simulink model "BPSK_modulation_demodulation_0"  (R2024a)
settings: Solver=VariableStepAuto  StartTime=0.0  StopTime=0.1  RelTol=1e-3
undefined symbols (not defined in the file or in its folder): Fs, ip, usb
libraries: commdigbbndpm3 x3, dspfdesign x3, commrflib2 x3, commfilt2 x3, dspsigops x3, plutoradiolib x1, simulink x1, dspxfrm3 x1, sdrrlib x1
settings Model: Creator=opr  LastModifiedBy=digital

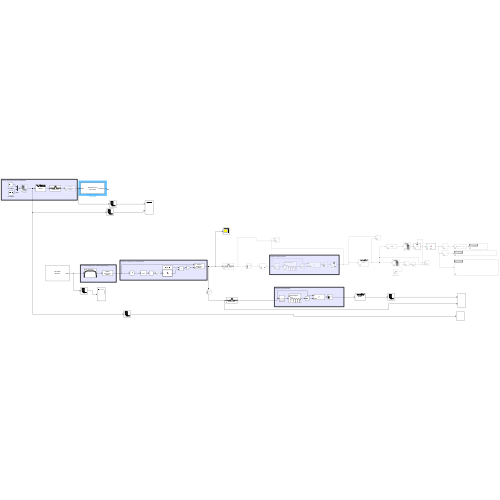
[thumbnail: Simulink's stored preview of the top-level diagram]
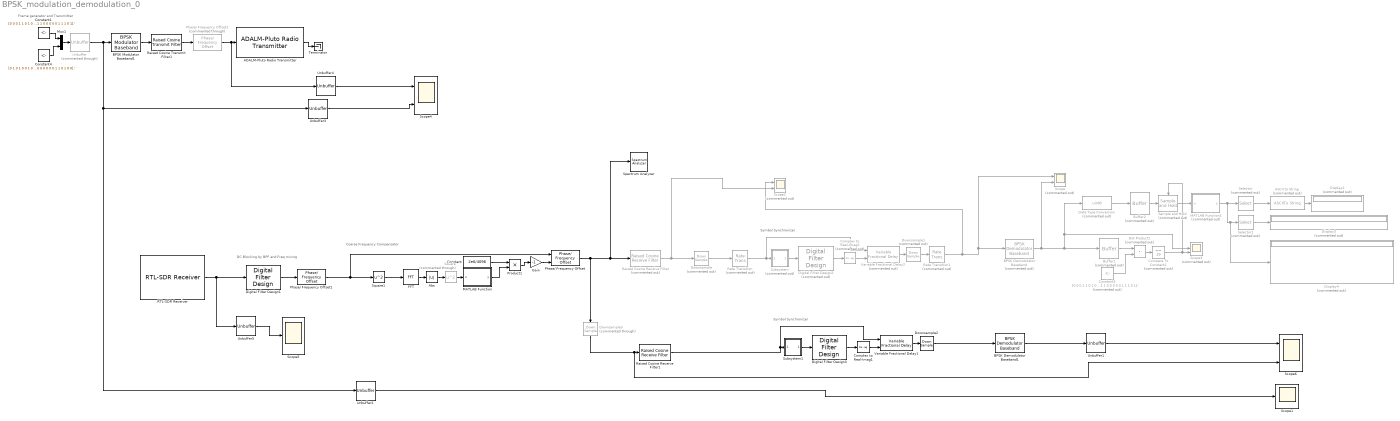
== system BPSK_modulation_demodulation_0 ==
  note: Coarse Frequency Compensator
  note: Frame generator and Transmitter
  note: DC Blocking by BPF and Freq mixing
  note: Symbol Synchronizer
  note: Symbol Synchronizer
  ADALM-Pluto Radio Transmitter : plutoradiolib/ADALM-Pluto Radio Transmitter  RadioID=usb:0  uri=ip:10.0.0.200  CenterFrequencySource=Dialog  CenterFrequency=450e6  GainSource=Dialog  Gain=-30  ChannelMapping=1  BasebandSampleRate=2e6  UnderflowOutputPort=on  ShowAdvancedProperties=off  UseCustomFilter=off  filtPathRates=[737280000 11520000 3840000 1920000 960000 240000]  filtCoefficients=[-192 82 85 -215 228 -102 -110 290 -318 145 160 -426 471 -215 -238 633 -697 318 349 -923 1009 -457 -498 1309 -1423 640 693 -1812 1959 -876 -945 2458 -2647 1180 1268 -3290 3534 -1572 -1688 4375 -4698 2091 2247 -5836 6284 -2807 -3031 7918 -8588 3870 4225 -11182 12324 -5662 -6330 17255 -19735 9507 11312 -33568 43355 -25227 -42139 305542 305542 -42139 -25227 43355 -33568 11312 9507 -19735 17255 -6330 -5662 12324 -11182 4225 3870 -8588 7918 -3031 -2807 6284 -5836 2247 2091 -4698 4375 -1688 -1572 3534 -3290 1268 1180 -2647 2458 -945 -876 1959 -1812 693 640 -1423 1309 -498 -457 1009 -923 349 318 -697 633 -238 -215 471 -426 160 145 -318 290 -110 -102 228 -215 85 82 -192]  filtCoefficientSize=128  filtDecimInterpFactor=4  filtGain=-12  filtRFBandwidth=18000000  filterConfigStruct=struct()  DataSourceSelect=Input Port  DDSTone1Freq=5e3  DDSTone2Freq=10e3  DDSTone1Scale=0.5  DDSTone2Scale=0.25  DataTimeout=Inf  FrequencyCorrection=0  ENSMPinControlMode=None  BISTLoopbackMode=Disabled  BISTToneInject=Disabled  BISTSignalGen=PRBS  BISTToneFreq=Fs/32  BISTToneLevel=0
  ASCII to String : ASCIIToString  Commented=on
  Abs : Abs  SaturateOnIntegerOverflow=off
  BPSK Demodulator Baseband : commdigbbndpm3/BPSK Demodulator Baseband  Commented=on  DecType=Hard decision  VarSource=Dialog  Variance=1  Ph=0  outDtype=Inherit via internal rule  derotateFactorWordLen=16  derotateFactorDataTypeStr=Inherit: Same word length as input  derotateFactorLastDataTypeStr=Inherit: Same word length as input
  BPSK Demodulator Baseband1 : commdigbbndpm3/BPSK Demodulator Baseband  DecType=Hard decision  VarSource=Dialog  Variance=1  Ph=0  outDtype=Inherit via internal rule  derotateFactorWordLen=16  derotateFactorDataTypeStr=Inherit: Same word length as input  derotateFactorLastDataTypeStr=Inherit: Same word length as input
  BPSK Modulator Baseband1 : commdigbbndpm3/BPSK Modulator Baseband  Ph=0  outDtype=double  outWordLen=16  outUDDataType=sfix(16)  outFracLenMode=Best precision  outFracLen=15  outDataTypeStr=double  outLastDataTypeStr=double
  Buffer1 : Buffer  Commented=on  N=32  V=31  OutputFrames=off
  Buffer2 : Buffer  Commented=on  N=160  V=159  OutputFrames=off
  Compare To Constant1 : simulink/Logic and Bit Operations/Compare To Constant  Commented=on  relop===  const=19  OutDataTypeStr=uint8
  Complex to Real-Imag1 : ComplexToRealImag  Output=Real
  Complex to Real-Imag2 : ComplexToRealImag  Commented=on  Output=Real
  Constant : Constant  Value=2e6/4096
  Constant1 : Constant  Value=[0 0 0 1 1 0 1 0 1 1 0 0 1 1 1 1 1 1 1 1 1 1 0 0 0 0 0 1 1 1 0 1].'  VectorParams1D=off  OutDataTypeStr=double  SampleTime=128/100e3
  Constant3 : Constant  Commented=on  Value=[0 0 0 1 1 0 1 0 1 1 0 0 1 1 1 1 1 1 1 1 1 1 0 0 0 0 0 1 1 1 0 1].'  VectorParams1D=off  OutDataTypeStr=double  SampleTime=1/10e6
  Constant4 : Constant  Value=[0 1 0 1 0 0 1 0 0 1 0 0 1 0 0 1 0 1 0 1 0 0 1 1 0 1 0 0 1 0 0 0 0 1 0 0 1 0 0 1 0 0 1 1 1 0 0 1 0 0 1 1 0 0 0 1 0 0 1 1 0 0 0 1 0 0 1 1 0 0 1 0 0 0 1 1 0 0 0 0 0 0 1 1 0 0 0 0 0 0 1 1 0 1 0 0].'  VectorParams1D=off  OutDataTypeStr=double  SampleTime=128/100e3
  Data Type Conversion : DataTypeConversion  Commented=on  OutDataTypeStr=uint8  SaturateOnIntegerOverflow=off  RndMeth=Floor
  Digital Filter Design1 : dspfdesign/Digital Filter Design  mwdsp_browser_bugfix_var=off
  Digital Filter Design2 : dspfdesign/Digital Filter Design  Commented=on  mwdsp_browser_bugfix_var=off
  Digital Filter Design3 : dspfdesign/Digital Filter Design  mwdsp_browser_bugfix_var=off
  Display2 : Display  Commented=on
  Display3 : Display  Commented=on
      settings: Format=hex (Stored Integer)
  Display4 : Display  Commented=on
      settings: Format=hex (Stored Integer)
  Dot Product1 : DotProduct  Commented=on  OutDataTypeStr=Inherit: Inherit via internal rule
  Downsample : DownSample  Commented=on  N=100  RateOptions=Allow multirate processing  AllowArbitraryFixedInput=on
  Downsample1 : DownSample  Commented=on  RateOptions=Allow multirate processing  AllowArbitraryFixedInput=on
  Downsample2 : DownSample  RateOptions=Allow multirate processing  AllowArbitraryFixedInput=on
  Downsample3 : DownSample  Commented=through  N=100  RateOptions=Allow multirate processing  AllowArbitraryFixedInput=on
  FFT : dspxfrm3/FFT  FFTImplementation=Auto  CompMethod=Table lookup  TableOpt=NEW  TableOptActive=Speed  BitRevOrder=off  Normalize=off  InheritFFTLength=on  FFTLength=64  WrapInput=on  roundingMode=Ceiling  overflowMode=off  firstCoeffDataTypeStr=Inherit: Same word length as input  firstCoeffLastDataTypeStr=Inherit: Same word length as input  outputMin=[]  outputMax=[]
  Gain : Gain  Gain=-1
  MATLAB Function : MATLAB Function  TreatAsAtomicUnit=on
  MATLAB Function1 : MATLAB Function  Commented=on  TreatAsAtomicUnit=on
  Mux1 : Mux  Inputs=2
  Phase/ Frequency Offset : commrflib2/Phase// Frequency Offset  phaseOffset=0  freqPort=on  freqOffset=0
  Phase/ Frequency Offset1 : commrflib2/Phase// Frequency Offset  phaseOffset=0  freqPort=off  freqOffset=-500e3
  Phase/ Frequency Offset2 : commrflib2/Phase// Frequency Offset  Commented=through  phaseOffset=0  freqPort=off  freqOffset=-500e3
  Product1 : Product
  RTL-SDR Receiver : sdrrlib/RTL-SDR Receiver  IPAddress=0  CenterFrequencySource=Dialog  CenterFrequency=449.5e6  GainSource=Dialog  Gain=20  ADCRate=2e6  FrequencyCorrection=0  LostSamplesOutputPort=off  LatencyOutputPort=off  OutputDataType=double  FrameLength=4096  EnableBurstMode=off  NumFramesInBurst=50  sobjType=sdrr.internal.SDRRTLReceiverSL  dataUDPPort=-1  ctrlUDPPort=-1  subDeviceList=nosubdev  sdrBlockType=SDRBlockTypeSLT.SDRRxBlock  requester=UNUSED_BY_SFCN  sdrExecutionMode=SDRExecutionModeSLT.ExecModeHW  BypassUserLogic=off  DecimatorSelect=DDC decimator  SourceSelect=RF data  SineAmplitude=16000  EnableInternalClock=off  BypassIQBalance=off  IFBandwidth=40e6  ADCRateSource=Dialog  IntermediateFrequency=0  DecimationFactorSource=Dialog  DecimationFactor=512  RFFrequencyIsTunable=logical(0)  SampleTime=(4096)/(2e6)  IFBandwidthSource=Dialog  SineFrequency=30000  BypassDCBlockingFilter=off  IntermediateFrequencySource=Dialog  IQBalanceCoefficients=64  SkipAllHardwareResetAndInitialization=off  EnableIQCalibrationTable=on  CacheIQCalibrationTable=off  EnableOffsetTuning=off  EnableRTLAGC=off  EnableTestMode=off  EnableTunerAGC=off  FrequencyCorrectionSource=Dialog  NumMLBuffers=128  NumUSBBuffers=16  RTLCrystalFrequency=28800000  TunerCrystalFrequency=28800000
  Raised Cosine Receive Filter : commfilt2/Raised Cosine Receive Filter  Commented=on  filtType=Square root  R=0.2  filtSpan=10  N=16  downFactor=8  downOffset=0  filterGain=1  RateOptions=Allow multirate processing  framing=Mute  checkCoeff=off  variableName=rcRxFilt  currentFiltSpan=10  D=5  inputOffset=0  sampMode=Mute  saveAsFlag=0  rateMode=Downsampling  checkGain=Normalized  launchFVT=on  roundingMode=Floor  overflowMode=off  coeffDataTypeStr=Inherit: Same word length as input  coeffMin=[]  coeffMax=[]  coeffLastDataTypeStr=Inherit: Same word length as input  accumDataTypeStr=Inherit: Same as product output  accumLastDataTypeStr=Inherit: Same as product output  outputDataTypeStr=Inherit: Same as accumulator  outputMin=[]  outputMax=[]  outputLastDataTypeStr=Inherit: Same as accumulator
  Raised Cosine Receive Filter1 : commfilt2/Raised Cosine Receive Filter  filtType=Square root  R=0.2  filtSpan=10  N=16  downFactor=8  downOffset=0  filterGain=1  InputProcessing=Columns as channels (frame based)  RateOptions=Allow multirate processing  framing=Mute  checkCoeff=off  variableName=rcRxFilt1  currentFiltSpan=10  D=5  inputOffset=0  sampMode=Mute  saveAsFlag=0  rateMode=Downsampling  checkGain=Normalized  launchFVT=on  roundingMode=Floor  overflowMode=off  coeffDataTypeStr=Inherit: Same word length as input  coeffMin=[]  coeffMax=[]  coeffLastDataTypeStr=Inherit: Same word length as input  accumDataTypeStr=Inherit: Same as product output  accumLastDataTypeStr=Inherit: Same as product output  outputDataTypeStr=Inherit: Same as accumulator  outputMin=[]  outputMax=[]  outputLastDataTypeStr=Inherit: Same as accumulator
  Raised Cosine Transmit Filter1 : commfilt2/Raised Cosine Transmit Filter  filtType=Square root  R=0.2  filtSpan=10  N=16  filterGain=1  InputProcessing=Columns as channels (frame based)  RateOptions=Allow multirate processing  framing=Mute  checkCoeff=off  variableName=rcTxFilt1  checkGain=Normalized  sampMode=Mute  saveAsFlag=0  currentFiltSpan=10  D=(10)/2  launchFVT=on  roundingMode=Floor  overflowMode=off  coeffDataTypeStr=Inherit: Same word length as input  coeffMin=[]  coeffMax=[]  coeffLastDataTypeStr=Inherit: Same word length as input  outputDataTypeStr=Inherit: Same as accumulator  outputMin=[]  outputMax=[]  outputLastDataTypeStr=Inherit: Same as accumulator
  Rate Transition : RateTransition  Commented=on  OutPortSampleTime=1/2e3
  Rate Transition1 : RateTransition  Commented=on  OutPortSampleTime=1/1e3
  Sample and Hold : dspsigops/Sample and Hold  Commented=on  trig=Rising edge  initCond=0  latchinput=off
  Scope : Scope  Commented=on  NumInputPorts=2
  Scope1 : Scope
  Scope2 : Scope  Commented=on  NumInputPorts=2
  Scope3 : Scope  Commented=on  NumInputPorts=3
  Scope4 : Scope  NumInputPorts=2
  Scope5 : Scope
  Scope6 : Scope  NumInputPorts=2
  Selector : Selector  Commented=on  NumberOfDimensions=2  InputPortWidth=3  IndexOptions=Index vector (dialog),Index vector (dialog)  Indices=[1: 12],1  OutputSizes=1,1
  Selector1 : Selector  Commented=on  NumberOfDimensions=2  InputPortWidth=3  IndexOptions=Index vector (dialog),Index vector (dialog)  Indices=[13:16],1  OutputSizes=1,1
  Spectrum Analyzer : SpectrumAnalyzer  WindowPosition=[0.000000,36.000000,2048.000000,1080.000000,]  ScopeFrameLocation=window  Span=2000000  StartFrequency=-1000000  StopFrequency=1000000  YLimits=[-81.07364636,-27.60033048]  SelectedToolstripTab=spectrumAnalyzerToolstrip.measurementsTab
  Square : Math  Commented=through  Operator=square
  Square1 : Math  Operator=square
  Subsystem : Subsystem  Commented=on
  Subsystem1 : Subsystem
  Terminator : Terminator
  Unbuffer : Unbuffer  Commented=through
  Unbuffer{1..5} (5 alike) : Unbuffer
  Variable Fractional Delay1 : dspsigops/Variable Fractional Delay  mode=OBSOLETE  modeActive=Linear  L=4  FarrowL=4  R=10  alpha=1  dmax=100  InputProcessing=Columns as channels (frame based)  ic=0  noDFT=off  fallbackFIR=Clip to the minimum value necessary for centered kernel  fallbackFarrow=Clip to the minimum value necessary for centered kernel  roundingMode=Zero  overflowMode=off
  Variable Fractional Delay2 : dspsigops/Variable Fractional Delay  Commented=on  mode=OBSOLETE  modeActive=Linear  L=4  FarrowL=4  R=10  alpha=1  dmax=100  ic=0  noDFT=off  fallbackFIR=Clip to the minimum value necessary for centered kernel  fallbackFarrow=Clip to the minimum value necessary for centered kernel  roundingMode=Zero  overflowMode=off
  wires:
  Downsample2/1 -> BPSK Demodulator Baseband1/1
  Selector1/1 -> Display3/1
  Square1/1 -> FFT/1
  Digital Filter Design1/1 -> Phase/ Frequency Offset1/1
  Raised Cosine Transmit Filter1/1 -> Phase/ Frequency Offset2/1
  Complex to Real-Imag2/1 -> Variable Fractional Delay2/2
  Constant1/1 -> Mux1/1
  Variable Fractional Delay1/1 -> Downsample2/1
  BPSK Demodulator Baseband/1 -> Scope/2, Data Type Conversion/1, Scope3/2, Buffer1/1
  Data Type Conversion/1 -> Buffer2/1
  Digital Filter Design3/1 -> Complex to Real-Imag1/1
  Phase/ Frequency Offset1/1 -> Square1/1, Phase/ Frequency Offset/1
  Product1/1 -> Gain/1
  Phase/ Frequency Offset2/1 -> Unbuffer4/1, ADALM-Pluto Radio Transmitter/1
  BPSK Modulator Baseband1/1 -> Raised Cosine Transmit Filter1/1
  Square/1 -> MATLAB Function/1(u)
  Rate Transition1/1 -> Scope2/1, Scope/1, BPSK Demodulator Baseband/1
  Raised Cosine Receive Filter/1 -> Downsample/1, Scope2/2
  ADALM-Pluto Radio Transmitter/1 -> Terminator/1
  Abs/1 -> Square/1
  Variable Fractional Delay2/1 -> Downsample1/1
  Downsample1/1 -> Rate Transition1/1
  Rate Transition/1 -> Variable Fractional Delay2/1, Subsystem/1(In2)
  Constant/1 -> Product1/1
  Constant3/1 -> Dot Product1/2
  Compare To Constant1/1 -> Sample and Hold/Trigger, Scope3/3
  RTL-SDR Receiver/1 -> Unbuffer5/1, Digital Filter Design1/1
  Dot Product1/1 -> Compare To Constant1/1
  Sample and Hold/1 -> MATLAB Function1/1(u)
  Downsample/1 -> Rate Transition/1
  Selector/1 -> ASCII to String/1
  Raised Cosine Receive Filter1/1 -> Variable Fractional Delay1/1, Subsystem1/1(In2)
  Buffer1/1 -> Dot Product1/1
  MATLAB Function/1(y) -> Product1/2
  Digital Filter Design2/1 -> Complex to Real-Imag2/1
  Complex to Real-Imag1/1 -> Variable Fractional Delay1/2
  FFT/1 -> Abs/1
  Gain/1 -> Phase/ Frequency Offset/2
  Constant4/1 -> Mux1/2
  Subsystem1/1(Out1) -> Digital Filter Design3/1
  Buffer2/1 -> Sample and Hold/1
  Mux1/1 -> Unbuffer/1
  Subsystem/1(Out1) -> Digital Filter Design2/1
  ASCII to String/1 -> Display2/1
  MATLAB Function1/1(y) -> Display4/1, Selector1/1, Selector/1
  BPSK Demodulator Baseband1/1 -> Unbuffer1/1
  Unbuffer2/1 -> Scope1/1
  Unbuffer1/1 -> Scope6/1
  Phase/ Frequency Offset/1 -> Downsample3/1, Spectrum Analyzer/1, Raised Cosine Receive Filter/1
  Downsample3/1 -> Scope6/2, Raised Cosine Receive Filter1/1
  Unbuffer/1 -> Unbuffer3/1, Unbuffer2/1, BPSK Modulator Baseband1/1
  Unbuffer3/1 -> Scope4/2
  Unbuffer4/1 -> Scope4/1
  Unbuffer5/1 -> Scope5/1

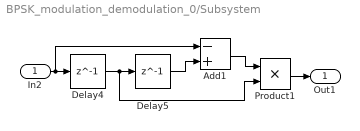
== system BPSK_modulation_demodulation_0/Subsystem ==
  In2 : Inport
  Add1 : Sum  Inputs=-+
  Delay4 : Delay  DelayLength=1  InitialCondition=0
  Delay5 : Delay  DelayLength=1  InitialCondition=0
  Product1 : Product
  Out1 : Outport
  wires:
  Add1/1 -> Product1/1
  In2/1 -> Add1/1, Delay4/1
  Delay5/1 -> Add1/2
  Delay4/1 -> Product1/2, Delay5/1
  Product1/1 -> Out1/1

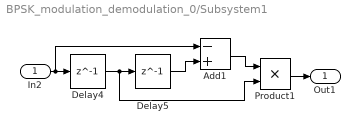
== system BPSK_modulation_demodulation_0/Subsystem1 ==
  In2 : Inport
  Add1 : Sum  Inputs=-+
  Delay4 : Delay  DelayLength=1  InitialCondition=0  InputProcessing=Columns as channels (frame based)
  Delay5 : Delay  DelayLength=1  InitialCondition=0  InputProcessing=Columns as channels (frame based)
  Product1 : Product
  Out1 : Outport
  wires:
  Add1/1 -> Product1/1
  In2/1 -> Add1/1, Delay4/1
  Delay5/1 -> Add1/2
  Delay4/1 -> Product1/2, Delay5/1
  Product1/1 -> Out1/1

== matlab function BPSK_modulation_demodulation_0/MATLAB Function ==
  data: u input; y output
function y = fcn(u)

[M,y] = max(u);

== matlab function BPSK_modulation_demodulation_0/MATLAB Function1 ==
  data: u input; y output
function y = fcn(u)
byte_matrix=reshape(u,8,[])';
y =bi2de(byte_matrix, 'left-msb');
